simulink model "TENG_switch_rectifier_converter"  (R2016a)
settings: Solver=VariableStepAuto  StartTime=0.0  StopTime=10.0  RelTol=1e-3
libraries: elec_lib x13, fl_lib x5, nesl_utility x3, simulink x1
settings Model: Creator=mugino  LastModifiedBy=mugino

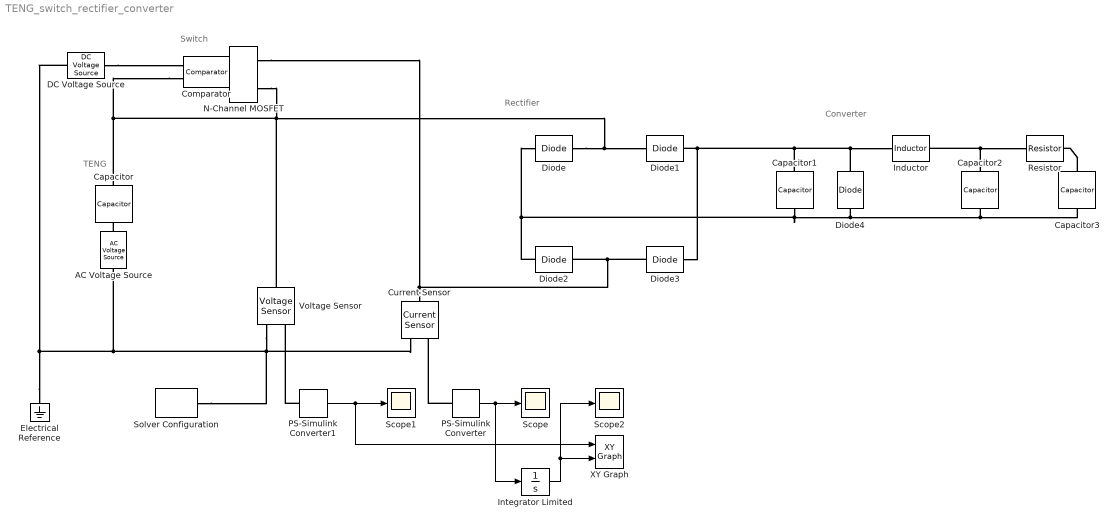
== system TENG_switch_rectifier_converter ==
  note: Rectifier
  note: Switch
  note: Converter
  note: TENG
  AC Voltage Source : fl_lib/Electrical/Electrical Sources/AC Voltage Source  amp=150 V  shift=0 deg  frequency=1 Hz  omega=0 rad/s
  Capacitor : elec_lib/Passive Devices/Capacitor  enable_table=0  c=1e-6 F  Cvec=[ 1e-5 1e-6 ] F  Vvec=[ 0 10 ] V  CV_table_symmetry=1  C_tol=5  enable_C_tol=0  tol_distribution=1  nSigma=4  r=60 MOhm  g=0 1/Ohm  initV=0 V  enable_operating_limits=0  operating_limit_action=2  max_working_voltage_range=[ -25 25 ] V  power_rating=1 W  enable_faults=0  fault_action=1  Cscale_faulted=100  R_faulted=0.001 Ohm  G_faulted=0 1/Ohm  tau_fault=0.001 s  enable_temporal_fault=0  t_fault=1 s  enable_behavioral_fault=0  max_permissible_voltage_range=[ -100 100 ] V  t_fail_on_voltage=1 s
  Capacitor1 : elec_lib/Passive Devices/Capacitor  enable_table=0  c=1e-6 F  Cvec=[ 1e-5 1e-6 ] F  Vvec=[ 0 10 ] V  CV_table_symmetry=1  C_tol=5  enable_C_tol=0  tol_distribution=1  nSigma=4  r=1e-6 MOhm  g=0 1/Ohm  initV=0 V  enable_operating_limits=0  operating_limit_action=2  max_working_voltage_range=[ -25 25 ] V  power_rating=1 W  enable_faults=0  fault_action=1  Cscale_faulted=100  R_faulted=0.001 Ohm  G_faulted=0 1/Ohm  tau_fault=0.001 s  enable_temporal_fault=0  t_fault=1 s  enable_behavioral_fault=0  max_permissible_voltage_range=[ -100 100 ] V  t_fail_on_voltage=1 s
  Capacitor2 : elec_lib/Passive Devices/Capacitor  enable_table=0  c=1e-6 F  Cvec=[ 1e-5 1e-6 ] F  Vvec=[ 0 10 ] V  CV_table_symmetry=1  C_tol=5  enable_C_tol=0  tol_distribution=1  nSigma=4  r=1e-6 MOhm  g=0 1/Ohm  initV=0 V  enable_operating_limits=0  operating_limit_action=2  max_working_voltage_range=[ -25 25 ] V  power_rating=1 W  enable_faults=0  fault_action=1  Cscale_faulted=100  R_faulted=0.001 Ohm  G_faulted=0 1/Ohm  tau_fault=0.001 s  enable_temporal_fault=0  t_fault=1 s  enable_behavioral_fault=0  max_permissible_voltage_range=[ -100 100 ] V  t_fail_on_voltage=1 s
  Capacitor3 : elec_lib/Passive Devices/Capacitor  enable_table=0  c=1e-6 F  Cvec=[ 1e-5 1e-6 ] F  Vvec=[ 0 10 ] V  CV_table_symmetry=1  C_tol=5  enable_C_tol=0  tol_distribution=1  nSigma=4  r=1e-6 Ohm  g=0 1/Ohm  initV=0 V  enable_operating_limits=0  operating_limit_action=1  max_working_voltage_range=[ -25 25 ] V  power_rating=1 W  enable_faults=0  fault_action=1  Cscale_faulted=100  R_faulted=0.001 Ohm  G_faulted=0 1/Ohm  tau_fault=0.001 s  enable_temporal_fault=0  t_fault=1 s  enable_behavioral_fault=0  max_permissible_voltage_range=[ -100 100 ] V  t_fail_on_voltage=1 s
  Comparator : elec_lib/Integrated Circuits/Comparator  V_OS=5 V  V_OL=0 V  V_OH=5 V  C_IN=0 pF  R_OUT=50 Ohm  Delay=0 s
  Current Sensor : fl_lib/Electrical/Electrical Sensors/Current Sensor
  DC Voltage Source : fl_lib/Electrical/Electrical Sources/DC Voltage Source  v0=140 V
  Diode{,1..4} (5 alike) : elec_lib/Semiconductor Devices/Diode  ModelType=1  Vf=0.6 V  Ron=0.3 Ohm  Goff=1e-8 S  Rz=0.3 Ohm  Vz=50 V  C_PWL=5 pF  prmExp=1  I12=[ 0.0137 0.545 ] A  V12=[ 0.6 0.7 ] V  I1=0.0137 A  V1=0.6 V  RS=0.01 Ohm  IS=1e-12 A  Tmeas=25 degC  ec=1  BV=Inf V  C_param=1  CJ0=5 pF  VJ=1 V  Mgrad=0.5  Vvec=[ 0.1 10 100 ] V  Cvec=[ 3.5 1 0.4 ] pF  FC=0.5  Q_param=1  Irrm=-7.15 A  iF=4 A  didt=-750 A/us  trr=115 ns  TT=50 ns  tau=100 ns  T_param=1  IS_T2=1.25e-7 A  I1_T2=0.245 A  V1_T2=0.5 V  Tmeas2=125 degC  EG_param=1  EG=1.11 eV  XTI_param=1  XTI=3  dBVdT=0 V/K  Tdevice=25 degC  Rth=[ 0 10 ] K/W  thermal_mass_parameterization=1  thermal_mass=[ 0 1 ] J/K  thermal_time_constant=[ 0 10 ] s  thermal_mass_initial_temperatures=[ 25 25 ] degC
  Electrical Reference : fl_lib/Electrical/Electrical Elements/Electrical Reference
  Inductor : elec_lib/Passive Devices/Inductor  l=1e-6 H  L_tol=20  enable_L_tol=0  tol_distribution=1  nSigma=4  r=0 Ohm  g=1e-9 1/Ohm  initI=0 A  enable_operating_limits=0  operating_limit_action=1  max_working_current=1 A  power_rating=1 W  enable_faults=0  fault_action=1  lambdaPercent=50  k_faulted=0.9999 Ohm  turnsShort=0  openCct=0  groundShort=0  groundShortG=0 1/Ohm  tau_fault=0.001 s  enable_temporal_fault=0  t_fault=1 s  enable_behavioral_fault=0  max_permissible_voltage=100 V  n_fail_on_voltage=1  max_permissible_current=1 A  t_fail_on_current=1 s
  Integrator Limited : Integrator  LimitOutput=on  UpperSaturationLimit=1  LowerSaturationLimit=0
  N-Channel MOSFET : elec_lib/Semiconductor Devices/N-Channel MOSFET  parameterization=1  prmDatasheet=1  prmEquCoeff=1  Beta=5 A/V^2  Rds=0.025 Ohm  Id=6 A  Vgs=10 V  Vth=1.7 V  lam=0 1/V  Tmeas=25 degC  RS=1e-4 Ohm  RD=0.01 Ohm  C_param=1  C_GS=270 pF  C_GD=80 pF  C_DS=0 pF  C_iss=350 pF  C_rss=80 pF  C_oss=0 pF  C_GS_vec=[ 270 300 290 280 295 255 ] pF  C_GD_vec=[ 450 400 300 190 95 55 ] pF  C_DS_vec=[ 450 410 390 230 175 115 ] pF  C_iss_vec=[ 720 700 590 470 390 310 ] pF  C_rss_vec=[ 450 400 300 190 95 55 ] pF  C_oss_vec=[ 900 810 690 420 270 170 ] pF  C_Vds_vec=[ 0.1 0.3 1 3 10 30 ] V  charge_linearity_param=1  C_OX=200 pF  V_C_OX=-0.5 V  dVth_dT=-6 mV/K  Rds_T2=0.037 Ohm  Tmeas2=125 degC  BEXDatasheet=-1.5  BEXEquCoeff=-1.5  TdeviceDatasheet=25 degC  TdeviceEquCoeff=25 degC  Rth=[ 0 10 ] K/W  thermal_mass_parameterization=1  thermal_mass=[ 0 1 ] J/K  thermal_time_constant=[ 0 10 ] s  thermal_mass_initial_temperatures=[ 25 25 ] degC
  PS-Simulink Converter : nesl_utility/PS-Simulink Converter  PhysicalDomain=network_engine_domain  SubClassName=ps_output  LeftPortType=input  RightPortType=output  PseudoPeriodic=off  Frequencies=[]  Unit=A  AffineConversion=off
  PS-Simulink Converter1 : nesl_utility/PS-Simulink Converter  PhysicalDomain=network_engine_domain  SubClassName=ps_output  LeftPortType=input  RightPortType=output  PseudoPeriodic=off  Frequencies=[]  Unit=V  AffineConversion=off
  Resistor : elec_lib/Passive Devices/Resistor  R=500 kOhm  R_tol=5  enable_R_tol=0  tol_distribution=1  nSigma=4  enable_operating_limits=0  operating_limit_action=2  max_working_voltage=100 V  power_rating=1 W  enable_faults=0  fault_action=1  R_faulted=Inf Ohm  enable_temporal_fault=0  t_fault=1 s  enable_behavioral_fault=0  max_permissible_current=1 A  t_fail_on_current=1 s  noise_mode=0  sample_time=0.001 s  repeatability=1  auto_seed=2032760128  user_seed=0  Tdevice=25 degC  alpha=0.00393 1/K  Tmeas=25 degC  thermal_mass=100 J/K  initial_temperature=25 degC  power_derating_T1=70 degC  power_derating_T2=155 degC  operating_temperature_range_vec=[ -50 150 ] degC
  Scope : Scope
  Scope1 : Scope
  Scope2 : Scope
  Solver Configuration : nesl_utility/Solver Configuration  PhysicalDomain=network_engine_domain  SubClassName=solver  LeftPortType=input  RightPortType=generic  Accelerate=off  Tones=[]  Harmonics=[]  SimulateNoise=off  Profile=off  UseLocalSampling=off  EnableSwitchedLinearOptims=on  FrequencyDomain=off  UseCCode=off  RelTol=0.001  AbsTol=1e-06  MinStep=1e-09  ToWorkspace=off  RevertToSquareIcSolve=off  NumHomotopyIterations=100  PhasorMode=off  PhasorModeNumHarmonics=1  OverrideAbsTol=off  DoDC=off  ResidualTolerance=1e-09  UseLocalSolver=off  LocalSolverChoice=NE_BACKWARD_EULER_ADVANCER  LocalSolverSampleTime=0.001  DoFixedCost=off  MaxNonlinIter=3  MaxModeIter=2  LinearAlgebra=Sparse  DelaysMemoryBudget=1024  AutomaticFiltering=on  FilteringTimeConstant=0.001
  Voltage Sensor : fl_lib/Electrical/Electrical Sensors/Voltage Sensor
  XY Graph : simulink/Sinks/XY Graph  xmin=-1  xmax=1  ymin=-1  ymax=1  st=-1
  wires:
  PS-Simulink Converter/1 -> Integrator Limited/1, Scope/1
  PS-Simulink Converter1/1 -> XY Graph/1, Scope1/1
  Integrator Limited/1 -> XY Graph/2, Scope2/1
  connections:
  Electrical Reference/LConn1 -- DC Voltage Source/RConn1 -- AC Voltage Source/RConn1 -- Solver Configuration/RConn1 -- Voltage Sensor/RConn2 -- Current Sensor/RConn2
  Comparator/LConn1 -- Capacitor/LConn1 -- Voltage Sensor/LConn1 -- N-Channel MOSFET/RConn2 -- Diode/RConn1 -- Diode1/LConn1
  Diode2/RConn1 -- Diode3/LConn1 -- N-Channel MOSFET/RConn1 -- Current Sensor/LConn1
  Capacitor1/LConn1 -- Diode4/RConn1 -- Inductor/LConn1 -- Diode3/RConn1 -- Diode1/RConn1
  Capacitor1/RConn1 -- Capacitor3/RConn1 -- Capacitor2/RConn1 -- Diode4/LConn1 -- Diode/LConn1 -- Diode2/LConn1
  PS-Simulink Converter/LConn1 -- Current Sensor/RConn1
  PS-Simulink Converter1/LConn1 -- Voltage Sensor/RConn1
  Comparator/RConn1 -- N-Channel MOSFET/LConn1
  DC Voltage Source/LConn1 -- Comparator/LConn2
  AC Voltage Source/LConn1 -- Capacitor/RConn1
  Capacitor2/LConn1 -- Inductor/RConn1 -- Resistor/LConn1
  Capacitor3/LConn1 -- Resistor/RConn1
